simulink model "test"  (R2016b)
settings: Solver=VariableStepAuto  StartTime=0.0  StopTime=10.0  RelTol=1e-3
values from neighbouring files (symbols this model uses):
  c = 400    [Active_Body_Control_param_stud.m]
  Km = 1    [Active_Body_Control_param_stud.m]
  L = 1e-5    (= 1e-05)    [Active_Body_Control_param_stud.m]
  m_va = 0.1    [Active_Body_Control_param_stud.m]
  R = 1.2    [Active_Body_Control_param_stud.m]
  s_max_va = 0.020    (= 0.02)    [Active_Body_Control_param_stud.m]
settings Model: Creator=ti.unbehaun  LastModifiedBy=ti.unbehaun

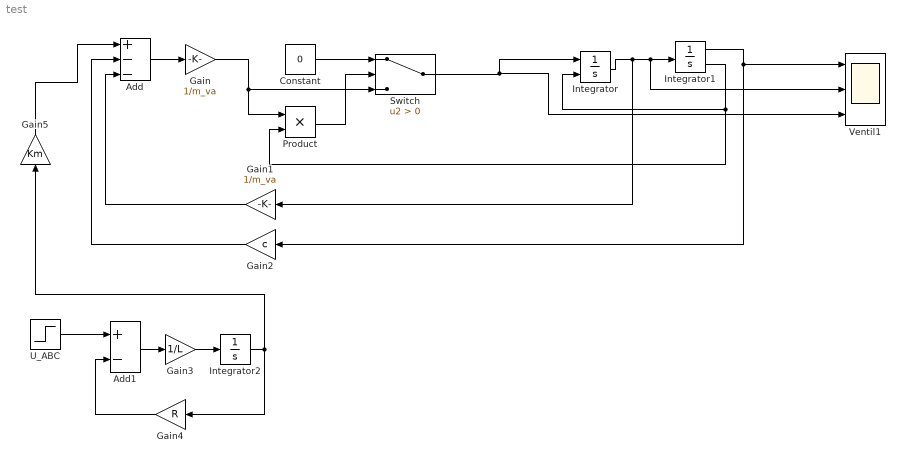
== system test ==
  Add : Sum  Inputs=+--
  Add1 : Sum  Inputs=+-
  Constant : Constant  Value=0
  Gain : Gain  Gain=1/m_va
  Gain1 : Gain  Gain=1/m_va
  Gain2 : Gain  Gain=c
  Gain3 : Gain  Gain=1/L
  Gain4 : Gain  Gain=R
  Gain5 : Gain  Gain=Km
  Integrator : Integrator  ExternalReset=either
  Integrator1 : Integrator  LimitOutput=on  UpperSaturationLimit=s_max_va  LowerSaturationLimit=-s_max_va  ShowSaturationPort=on
  Integrator2 : Integrator
  Product : Product
  Switch : Switch  Criteria=u2 > Threshold
  U_ABC : Step  Time=5  Before=20  After=-20  SampleTime=0
  Ventil1 : Scope  NumInputPorts=3
  wires:
  Add/1 -> Gain/1
  Gain/1 -> Switch/3, Product/1
  Integrator/1 -> Gain1/1, Ventil1/2, Integrator1/1
  Gain1/1 -> Add/3
  Integrator1/1 -> Ventil1/1, Gain2/1
  Gain2/1 -> Add/2
  Integrator2/1 -> Gain4/1, Gain5/1
  U_ABC/1 -> Add1/1
  Add1/1 -> Gain3/1
  Gain3/1 -> Integrator2/1
  Gain4/1 -> Add1/2
  Gain5/1 -> Add/1
  Integrator1/2 -> Product/2, Integrator/2
  Switch/1 -> Ventil1/3, Integrator/1
  Product/1 -> Switch/2
  Constant/1 -> Switch/1
